simulink model "FullCarLateral"  (R2023b)
settings: Solver=FixedStepAuto  StartTime=0.0  StopTime=30  FixedStep=dt  MaxStep=0.001  RelTol=1e-3
model workspace (MAT data in the model file):
  AMU : Simulink.Signal (value not decoded)
  EPSILON : Simulink.Signal (value not decoded)
  FZO : Simulink.Signal (value not decoded)
  LCX : Simulink.Signal (value not decoded)
  LCY : Simulink.Signal (value not decoded)
  LCZ : Simulink.Signal (value not decoded)
  LEX : Simulink.Signal (value not decoded)
  LEY : Simulink.Signal (value not decoded)
  LFZO : Simulink.Signal (value not decoded)
  LHX : Simulink.Signal (value not decoded)
  LHY : Simulink.Signal (value not decoded)
  LKXKAPPA : Simulink.Signal (value not decoded)
  LKYALPHA : Simulink.Signal (value not decoded)
  LKYGAMMA : Simulink.Signal (value not decoded)
  LKZGAMMA : Simulink.Signal (value not decoded)
  LMR : Simulink.Signal (value not decoded)
  LMUV : Simulink.Signal (value not decoded)
  LMUX : Simulink.Signal (value not decoded)
  LMUXAST : Simulink.Signal (value not decoded)
  LMUXPRIME : Simulink.Signal (value not decoded)
  LMUY : Simulink.Signal (value not decoded)
  LMUYAST : Simulink.Signal (value not decoded)
  LMUYPRIME : Simulink.Signal (value not decoded)
  LMX : Simulink.Signal (value not decoded)
  LMY : Simulink.Signal (value not decoded)
  LS : Simulink.Signal (value not decoded)
  LT : Simulink.Signal (value not decoded)
  LVX : Simulink.Signal (value not decoded)
  LVY : Simulink.Signal (value not decoded)
  LVYKAPPA : Simulink.Signal (value not decoded)
  LXALPHA : Simulink.Signal (value not decoded)
  LYKAPPA : Simulink.Signal (value not decoded)
  PCX1 : Simulink.Signal (value not decoded)
  PCY1 : Simulink.Signal (value not decoded)
  PDX1 : Simulink.Signal (value not decoded)
  PDX2 : Simulink.Signal (value not decoded)
  PDX3 : Simulink.Signal (value not decoded)
  PDY1 : Simulink.Signal (value not decoded)
  PDY2 : Simulink.Signal (value not decoded)
  PDY3 : Simulink.Signal (value not decoded)
  PEX1 : Simulink.Signal (value not decoded)
  PEX2 : Simulink.Signal (value not decoded)
  PEX3 : Simulink.Signal (value not decoded)
  PEX4 : Simulink.Signal (value not decoded)
  PEY1 : Simulink.Signal (value not decoded)
  PEY2 : Simulink.Signal (value not decoded)
  PEY3 : Simulink.Signal (value not decoded)
  PEY4 : Simulink.Signal (value not decoded)
  PEY5 : Simulink.Signal (value not decoded)
  PHX1 : Simulink.Signal (value not decoded)
  PHX2 : Simulink.Signal (value not decoded)
  PHY1 : Simulink.Signal (value not decoded)
  PHY2 : Simulink.Signal (value not decoded)
  PKX1 : Simulink.Signal (value not decoded)
  PKX2 : Simulink.Signal (value not decoded)
  PKX3 : Simulink.Signal (value not decoded)
  PKY1 : Simulink.Signal (value not decoded)
  PKY2 : Simulink.Signal (value not decoded)
  PKY3 : Simulink.Signal (value not decoded)
  PKY4 : Simulink.Signal (value not decoded)
  PKY5 : Simulink.Signal (value not decoded)
  PKY6 : Simulink.Signal (value not decoded)
  PKY7 : Simulink.Signal (value not decoded)
  PVX1 : Simulink.Signal (value not decoded)
  PVX2 : Simulink.Signal (value not decoded)
  PVY1 : Simulink.Signal (value not decoded)
  PVY2 : Simulink.Signal (value not decoded)
  PVY3 : Simulink.Signal (value not decoded)
  PVY4 : Simulink.Signal (value not decoded)
  QBZ1 : Simulink.Signal (value not decoded)
  QBZ10 : Simulink.Signal (value not decoded)
  QBZ2 : Simulink.Signal (value not decoded)
  QBZ3 : Simulink.Signal (value not decoded)
  QBZ5 : Simulink.Signal (value not decoded)
  QBZ6 : Simulink.Signal (value not decoded)
  QBZ9 : Simulink.Signal (value not decoded)
  QCZ1 : Simulink.Signal (value not decoded)
  QDZ1 : Simulink.Signal (value not decoded)
  QDZ10 : Simulink.Signal (value not decoded)
  QDZ11 : Simulink.Signal (value not decoded)
  QDZ2 : Simulink.Signal (value not decoded)
  QDZ3 : Simulink.Signal (value not decoded)
  QDZ4 : Simulink.Signal (value not decoded)
  QDZ6 : Simulink.Signal (value not decoded)
  QDZ7 : Simulink.Signal (value not decoded)
  QDZ8 : Simulink.Signal (value not decoded)
  QDZ9 : Simulink.Signal (value not decoded)
  QEZ1 : Simulink.Signal (value not decoded)
  QEZ2 : Simulink.Signal (value not decoded)
  QEZ3 : Simulink.Signal (value not decoded)
  QEZ4 : Simulink.Signal (value not decoded)
  QEZ5 : Simulink.Signal (value not decoded)
  QHZ1 : Simulink.Signal (value not decoded)
  QHZ2 : Simulink.Signal (value not decoded)
  QHZ3 : Simulink.Signal (value not decoded)
  QHZ4 : Simulink.Signal (value not decoded)
  QSX1 : Simulink.Signal (value not decoded)
  QSX2 : Simulink.Signal (value not decoded)
  QSX3 : Simulink.Signal (value not decoded)
  QX1 : Simulink.Signal (value not decoded)
  QX2 : Simulink.Signal (value not decoded)
  QX3 : Simulink.Signal (value not decoded)
  QX4 : Simulink.Signal (value not decoded)
  QX5 : Simulink.Signal (value not decoded)
  QX6 : Simulink.Signal (value not decoded)
  RBX1 : Simulink.Signal (value not decoded)
  RBX2 : Simulink.Signal (value not decoded)
  RBX3 : Simulink.Signal (value not decoded)
  RBY1 : Simulink.Signal (value not decoded)
  RBY2 : Simulink.Signal (value not decoded)
  RBY3 : Simulink.Signal (value not decoded)
  RBY4 : Simulink.Signal (value not decoded)
  RCX1 : Simulink.Signal (value not decoded)
  RCY1 : Simulink.Signal (value not decoded)
  REX1 : Simulink.Signal (value not decoded)
  REX2 : Simulink.Signal (value not decoded)
  REY1 : Simulink.Signal (value not decoded)
  REY2 : Simulink.Signal (value not decoded)
  RHX1 : Simulink.Signal (value not decoded)
  RHY1 : Simulink.Signal (value not decoded)
  RHY2 : Simulink.Signal (value not decoded)
  RO : Simulink.Signal (value not decoded)
  RVY1 : Simulink.Signal (value not decoded)
  RVY2 : Simulink.Signal (value not decoded)
  RVY3 : Simulink.Signal (value not decoded)
  RVY4 : Simulink.Signal (value not decoded)
  RVY5 : Simulink.Signal (value not decoded)
  RVY6 : Simulink.Signal (value not decoded)
  SSZ1 : Simulink.Signal (value not decoded)
  SSZ2 : Simulink.Signal (value not decoded)
  SSZ3 : Simulink.Signal (value not decoded)
  SSZ4 : Simulink.Signal (value not decoded)
  VCX : Simulink.Signal (value not decoded)
  ZETA0 : Simulink.Signal (value not decoded)
  ZETA1 : Simulink.Signal (value not decoded)
  ZETA2 : Simulink.Signal (value not decoded)
  ZETA3 : Simulink.Signal (value not decoded)
  ZETA4 : Simulink.Signal (value not decoded)
  ZETA5 : Simulink.Signal (value not decoded)
  ZETA6 : Simulink.Signal (value not decoded)
  ZETA7 : Simulink.Signal (value not decoded)
  ZETA8 : Simulink.Signal (value not decoded)
values from neighbouring files (symbols this model uses):
  A = load('PSS LATERAL FORCE COEFFS.mat').A    [FullCarLateralParams.m]
  B = load('PSS ALIGNING TORQUE COEFFS.mat').B    [FullCarLateralParams.m]
  b = 0.085    [FullCarLateralParams.m]
  C = load('COMBINED OVERTURNING MOMENT COEFFS.mat').C    [FullCarLateralParams.m]
  c_roll = 0.1    [FullCarLateralParams.m]
  cD = 1.23    [FullCarLateralParams.m]
  cL = 3.71    [FullCarLateralParams.m]
  D = load('PLS LONGITUDINAL FORCE COEFFS.mat').D    [FullCarLateralParams.m]
  dt = 0.001    [FullCarLateralParams.m]
  E = load('COMBINED LONGITUDINAL FORCE COEFFS.mat').E    [FullCarLateralParams.m]
  e_FL = atan(tf/lf)    [FullCarLateralParams.m]
  e_FR = atan(lf/tf)    [FullCarLateralParams.m]
  e_RL = atan(lr/tr)    [FullCarLateralParams.m]
  e_RR = atan(tr/lr)    [FullCarLateralParams.m]
  F = load('COMBINED LATERAL FORCE COEFFS.mat').F    [FullCarLateralParams.m]
  frontalA = 1    [FullCarLateralParams.m]
  g = 9.81    [FullCarLateralParams.m]
  G = load('COMBINED ALIGNING TORQUE COEFFS.mat').G    [FullCarLateralParams.m]
  gearboxEff = 0.95    [FullCarLateralParams.m]
  GR = 11.86    [FullCarLateralParams.m]
  hCG = 0.2    [FullCarLateralParams.m]
  Ix_wheel = (0.07829 + Ix_motor*GR*GR) * Ix_wheel_factor    (= 0.1168307304)    [FullCarLateralParams.m]
  Iz_vehicle = 125    [FullCarLateralParams.m]
  lf = wb - lr    (= 0.755)    [FullCarLateralParams.m]
  lowpassT = 0.05    [FullCarLateralParams.m]
  lr = 0.78    [FullCarLateralParams.m]
  m = 250    [FullCarLateralParams.m]
  motorOmegaLimit = 2094    [FullCarLateralParams.m]
  R_FL = sqrt(tf^2 + lf^2)    [FullCarLateralParams.m]
  R_FR = R_FL    [FullCarLateralParams.m]
  R_RL = sqrt(tr^2 + lr^2)    [FullCarLateralParams.m]
  R_RR = R_RL    [FullCarLateralParams.m]
  R_wheel = 0.2    [FullCarLateralParams.m]
  rho = 1.293    [FullCarLateralParams.m]
  tireFactor_X_Accel = 0.6    [FullCarLateralParams.m]
  tireFactor_X_Brake = 0.6    [FullCarLateralParams.m]
  tireFactor_Y = 1    [FullCarLateralParams.m]
  TLLTD = 0.5    [FullCarLateralParams.m]
  tr = trackWidth / 2    (= 0.6)    [FullCarLateralParams.m]
  trackWidth = 1.2    [FullCarLateralParams.m]
  wb = 1.535    [FullCarLateralParams.m]
  wheelSideBrakeFactor = 1    [FullCarLateralParams.m]
undefined symbols (not defined in the file or in its folder): trackReference
libraries: simulink_extras x11, eeGeneralControl x3, slpidlib x2, simulink x2
(part 4 of 6)

== system FullCarLateral/Car/Wheel Dynamics/Subsystem7/Accel. or Rolling No Slip ==
  Requested Motor Torque : Inport
  FX Resistance : Inport  Port=2
  Long Corner Vel : Inport  Port=3
  Action Port : ActionPort  ActionPortLabel=if(u1 >= 0)
  Accelerating : Subsystem  TreatAsAtomicUnit=on
  If : If  IfExpression=u1 > rollingNoSlipTorqueThreshold
  Merge : Merge
  Merge1 : Merge
  Rolling No Slip : Subsystem  TreatAsAtomicUnit=on
  Wheel Omega : Outport
  Constrained Motor Torque : Outport  Port=2
  wires:
  Merge1/1 -> Constrained Motor Torque/1
  Rolling No Slip/2(Constrained Motor Torque) -> Merge1/2
  Accelerating/2(Constrained Motor Torque) -> Merge1/1
  FX Resistance/1 -> Accelerating/2(FX Resistance)
  Long Corner Vel/1 -> Rolling No Slip/1(Long Corner Vel)
  Merge/1 -> Wheel Omega/1
  Rolling No Slip/1(No Slip Wheel Omega) -> Merge/2
  Accelerating/1(Accelerating Wheel Omega) -> Merge/1
  If/2 -> Rolling No Slip/Action
  If/1 -> Accelerating/Action
  Requested Motor Torque/1 -> If/1, Rolling No Slip/2(Requested Motor Torque), Accelerating/1(Requested Motor Torque)

== system FullCarLateral/Car/Wheel Dynamics/Subsystem7/Braking ==
  Requested Motor Torque : Inport
  FX Resistance : Inport  Port=2
  Action Port : ActionPort  ActionPortLabel=else
  Constant : Constant  Value=0
  Motor Omega Calc : Subsystem
  Switch : Switch  Criteria=u2 > Threshold  SaturateOnIntegerOverflow=off  InputSameDT=off
  Wheel Omega : Outport
  Constrained Motor Torque : Outport  Port=2
  wires:
  Constant/1 -> Switch/3
  Switch/1 -> Wheel Omega/1
  Motor Omega Calc/1(Wheel Omega) -> Switch/1, Switch/2
  FX Resistance/1 -> Motor Omega Calc/2(FX Resistance)
  Requested Motor Torque/1 -> Motor Omega Calc/1(Motor Torque), Constrained Motor Torque/1

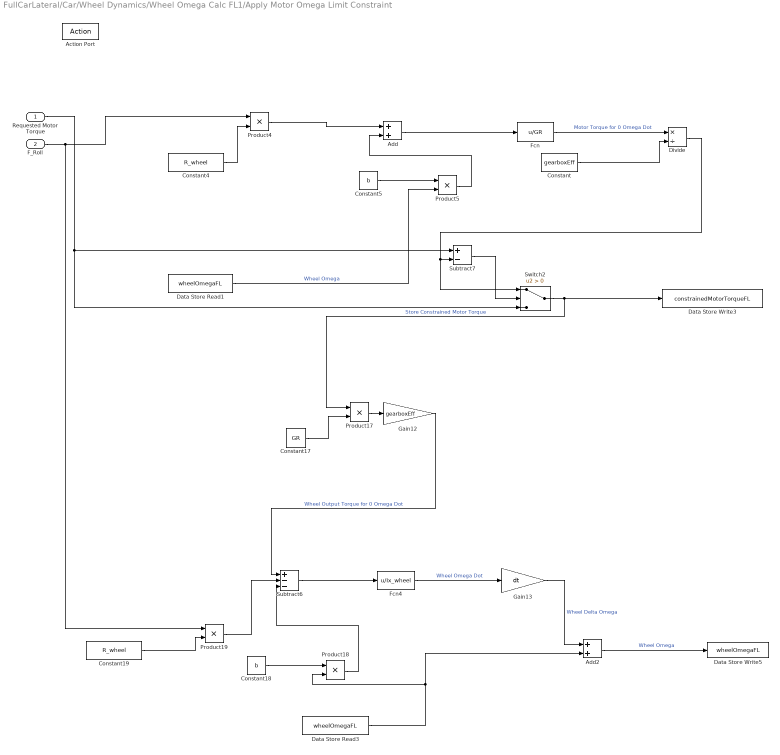
== system FullCarLateral/Car/Wheel Dynamics/Wheel Omega Calc FL1/Apply Motor Omega Limit Constraint ==
  Requested Motor Torque : Inport
  F_Roll : Inport  Port=2
  Action Port : ActionPort
  Add : Sum
  Add2 : Sum
  Constant : Constant  Value=gearboxEff
  Constant17 : Constant  Value=GR
  Constant18 : Constant  Value=b
  Constant19 : Constant  Value=R_wheel
  Constant4 : Constant  Value=R_wheel
  Constant5 : Constant  Value=b
  Data Store Read1 : DataStoreRead  DataStoreName=wheelOmegaFL  IndexOptions=Index vector (dialog)  Indices=1  OutputSizes=1
  Data Store Read3 : DataStoreRead  DataStoreName=wheelOmegaFL  IndexOptions=Index vector (dialog)  Indices=1  OutputSizes=1
  Data Store Write3 : DataStoreWrite  DataStoreName=constrainedMotorTorqueFL  IndexOptions=Index vector (dialog)  Indices=1  OutputSizes=1
  Data Store Write5 : DataStoreWrite  DataStoreName=wheelOmegaFL  IndexOptions=Index vector (dialog)  Indices=1  OutputSizes=1
  Divide : Product  Inputs=*/
  Fcn : Fcn  Expr=u/GR
  Fcn4 : Fcn  Expr=u/Ix_wheel
  Gain12 : Gain  Gain=gearboxEff
  Gain13 : Gain  Gain=dt
  Product{4..5,17..19} (5 alike) : Product
  Subtract6 : Sum  Inputs=+--
  Subtract7 : Sum  Inputs=+-
  Switch2 : Switch  Criteria=u2 > Threshold  SaturateOnIntegerOverflow=off  InputSameDT=off
  wires:
  Constant5/1 -> Product5/1
  Add/1 -> Fcn/1
  Constant4/1 -> Product4/2
  Product5/1 -> Add/2
  Product4/1 -> Add/1
  Switch2/1 -> Product17/1, Data Store Write3/1  "Store Constrained Motor Torque"
  Gain12/1 -> Subtract6/1  "Wheel Output Torque for 0 Omega Dot"
  Subtract7/1 -> Switch2/2
  Data Store Read3/1 -> Add2/2, Product18/2
  Constant18/1 -> Product18/1
  Requested Motor Torque/1 -> Subtract7/1, Switch2/3
  Product17/1 -> Gain12/1
  Fcn4/1 -> Gain13/1  "Wheel Omega Dot"
  Subtract6/1 -> Fcn4/1
  Product19/1 -> Subtract6/2
  Constant17/1 -> Product17/2
  Gain13/1 -> Add2/1  "Wheel Delta Omega"
  Product18/1 -> Subtract6/3
  Add2/1 -> Data Store Write5/1  "Wheel Omega"
  Constant19/1 -> Product19/2
  F_Roll/1 -> Product19/1, Product4/1
  Data Store Read1/1 -> Product5/2  "Wheel Omega"
  Fcn/1 -> Divide/1  "Motor Torque for 0 Omega Dot"
  Constant/1 -> Divide/2
  Divide/1 -> Switch2/1, Subtract7/2

== system FullCarLateral/Car/Wheel Dynamics/Wheel Omega Calc FL1/No Omega Limit Constraint ==
  Wheel Omega : Inport
  Unconstrained Requested Motor Torque : Inport  Port=2
  Action Port : ActionPort
  Constant1 : Constant  Value=0
  Data Store Write3 : DataStoreWrite  DataStoreName=constrainedMotorTorqueFL  IndexOptions=Index vector (dialog)  Indices=1  OutputSizes=1
  Data Store Write6 : DataStoreWrite  DataStoreName=wheelOmegaFL  IndexOptions=Index vector (dialog)  Indices=1  OutputSizes=1
  Switch : Switch  Criteria=u2 > Threshold  SaturateOnIntegerOverflow=off  InputSameDT=off
  wires:
  Unconstrained Requested Motor Torque/1 -> Data Store Write3/1
  Constant1/1 -> Switch/3
  Wheel Omega/1 -> Switch/1, Switch/2  "Wheel Omega"
  Switch/1 -> Data Store Write6/1

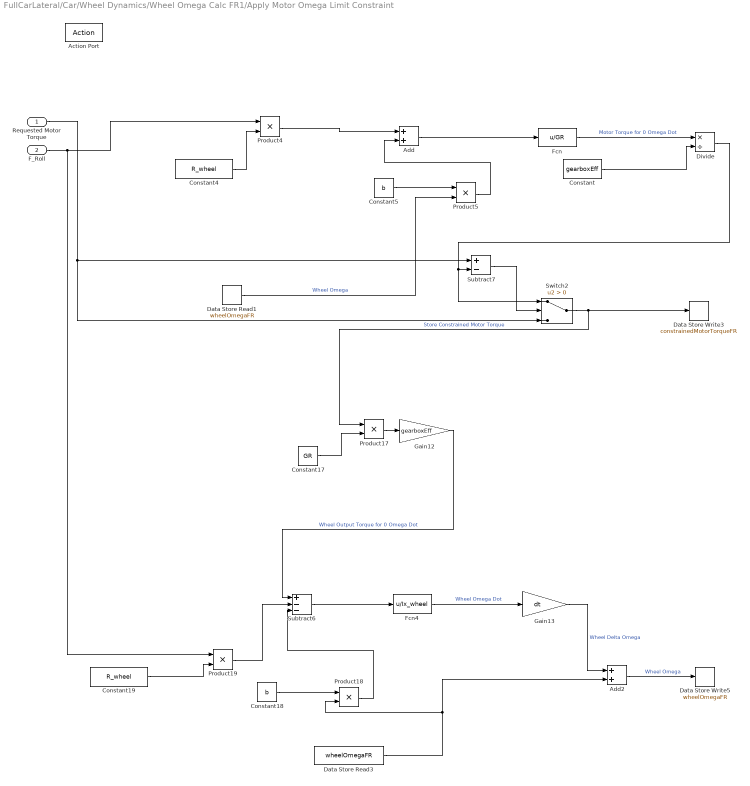
== system FullCarLateral/Car/Wheel Dynamics/Wheel Omega Calc FR1/Apply Motor Omega Limit Constraint ==
  Requested Motor Torque : Inport
  F_Roll : Inport  Port=2
  Action Port : ActionPort
  Add : Sum
  Add2 : Sum
  Constant : Constant  Value=gearboxEff
  Constant17 : Constant  Value=GR
  Constant18 : Constant  Value=b
  Constant19 : Constant  Value=R_wheel
  Constant4 : Constant  Value=R_wheel
  Constant5 : Constant  Value=b
  Data Store Read1 : DataStoreRead  DataStoreName=wheelOmegaFR  IndexOptions=Index vector (dialog)  Indices=1  OutputSizes=1
  Data Store Read3 : DataStoreRead  DataStoreName=wheelOmegaFR  IndexOptions=Index vector (dialog)  Indices=1  OutputSizes=1
  Data Store Write3 : DataStoreWrite  DataStoreName=constrainedMotorTorqueFR  IndexOptions=Index vector (dialog)  Indices=1  OutputSizes=1
  Data Store Write5 : DataStoreWrite  DataStoreName=wheelOmegaFR  IndexOptions=Index vector (dialog)  Indices=1  OutputSizes=1
  Divide : Product  Inputs=*/
  Fcn : Fcn  Expr=u/GR
  Fcn4 : Fcn  Expr=u/Ix_wheel
  Gain12 : Gain  Gain=gearboxEff
  Gain13 : Gain  Gain=dt
  Product{4..5,17..19} (5 alike) : Product
  Subtract6 : Sum  Inputs=+--
  Subtract7 : Sum  Inputs=+-
  Switch2 : Switch  Criteria=u2 > Threshold  SaturateOnIntegerOverflow=off  InputSameDT=off
  wires:
  Divide/1 -> Subtract7/2, Switch2/1
  Constant/1 -> Divide/2
  Fcn/1 -> Divide/1  "Motor Torque for 0 Omega Dot"
  Data Store Read1/1 -> Product5/2  "Wheel Omega"
  F_Roll/1 -> Product4/1, Product19/1
  Constant19/1 -> Product19/2
  Add2/1 -> Data Store Write5/1  "Wheel Omega"
  Product18/1 -> Subtract6/3
  Gain13/1 -> Add2/1  "Wheel Delta Omega"
  Constant17/1 -> Product17/2
  Product19/1 -> Subtract6/2
  Subtract6/1 -> Fcn4/1
  Fcn4/1 -> Gain13/1  "Wheel Omega Dot"
  Product17/1 -> Gain12/1
  Requested Motor Torque/1 -> Switch2/3, Subtract7/1
  Constant18/1 -> Product18/1
  Data Store Read3/1 -> Product18/2, Add2/2
  Subtract7/1 -> Switch2/2
  Gain12/1 -> Subtract6/1  "Wheel Output Torque for 0 Omega Dot"
  Switch2/1 -> Data Store Write3/1, Product17/1  "Store Constrained Motor Torque"
  Product4/1 -> Add/1
  Product5/1 -> Add/2
  Constant4/1 -> Product4/2
  Add/1 -> Fcn/1
  Constant5/1 -> Product5/1

== system FullCarLateral/Car/Wheel Dynamics/Wheel Omega Calc FR1/No Omega Limit Constraint ==
  Wheel Omega : Inport
  Unconstrained Requested Motor Torque : Inport  Port=2
  Action Port : ActionPort
  Constant1 : Constant  Value=0
  Data Store Write3 : DataStoreWrite  DataStoreName=constrainedMotorTorqueFR  IndexOptions=Index vector (dialog)  Indices=1  OutputSizes=1
  Data Store Write6 : DataStoreWrite  DataStoreName=wheelOmegaFR  IndexOptions=Index vector (dialog)  Indices=1  OutputSizes=1
  Switch : Switch  Criteria=u2 > Threshold  SaturateOnIntegerOverflow=off  InputSameDT=off
  wires:
  Unconstrained Requested Motor Torque/1 -> Data Store Write3/1
  Switch/1 -> Data Store Write6/1
  Wheel Omega/1 -> Switch/2, Switch/1  "Wheel Omega"
  Constant1/1 -> Switch/3

== system FullCarLateral/Car/Wheel Dynamics/Wheel Omega Calc RL1/Apply Motor Omega Limit Constraint ==
  Requested Motor Torque : Inport
  F_Roll : Inport  Port=2
  Action Port : ActionPort
  Add : Sum
  Add2 : Sum
  Constant : Constant  Value=gearboxEff
  Constant17 : Constant  Value=GR
  Constant18 : Constant  Value=b
  Constant19 : Constant  Value=R_wheel
  Constant4 : Constant  Value=R_wheel
  Constant5 : Constant  Value=b
  Data Store Read1 : DataStoreRead  DataStoreName=wheelOmegaRL  IndexOptions=Index vector (dialog)  Indices=1  OutputSizes=1
  Data Store Read3 : DataStoreRead  DataStoreName=wheelOmegaRL  IndexOptions=Index vector (dialog)  Indices=1  OutputSizes=1
  Data Store Write3 : DataStoreWrite  DataStoreName=constrainedMotorTorqueRL  IndexOptions=Index vector (dialog)  Indices=1  OutputSizes=1
  Data Store Write5 : DataStoreWrite  DataStoreName=wheelOmegaRL  IndexOptions=Index vector (dialog)  Indices=1  OutputSizes=1
  Divide : Product  Inputs=*/
  Fcn : Fcn  Expr=u/GR
  Fcn4 : Fcn  Expr=u/Ix_wheel
  Gain12 : Gain  Gain=gearboxEff
  Gain13 : Gain  Gain=dt
  Product{4..5,17..19} (5 alike) : Product
  Subtract6 : Sum  Inputs=+--
  Subtract7 : Sum  Inputs=+-
  Switch2 : Switch  Criteria=u2 > Threshold  SaturateOnIntegerOverflow=off  InputSameDT=off
  wires:
  Constant5/1 -> Product5/1
  Add/1 -> Fcn/1
  Constant4/1 -> Product4/2
  Product5/1 -> Add/2
  Product4/1 -> Add/1
  Switch2/1 -> Product17/1, Data Store Write3/1  "Store Constrained Motor Torque"
  Gain12/1 -> Subtract6/1  "Wheel Output Torque for 0 Omega Dot"
  Subtract7/1 -> Switch2/2
  Data Store Read3/1 -> Add2/2, Product18/2
  Constant18/1 -> Product18/1
  Requested Motor Torque/1 -> Subtract7/1, Switch2/3
  Product17/1 -> Gain12/1
  Fcn4/1 -> Gain13/1  "Wheel Omega Dot"
  Subtract6/1 -> Fcn4/1
  Product19/1 -> Subtract6/2
  Constant17/1 -> Product17/2
  Gain13/1 -> Add2/1  "Wheel Delta Omega"
  Product18/1 -> Subtract6/3
  Add2/1 -> Data Store Write5/1  "Wheel Omega"
  Constant19/1 -> Product19/2
  F_Roll/1 -> Product19/1, Product4/1
  Data Store Read1/1 -> Product5/2  "Wheel Omega"
  Fcn/1 -> Divide/1  "Motor Torque for 0 Omega Dot"
  Constant/1 -> Divide/2
  Divide/1 -> Switch2/1, Subtract7/2

== system FullCarLateral/Car/Wheel Dynamics/Wheel Omega Calc RL1/No Omega Limit Constraint ==
  Wheel Omega : Inport
  Unconstrained Requested Motor Torque : Inport  Port=2
  Action Port : ActionPort
  Constant1 : Constant  Value=0
  Data Store Write3 : DataStoreWrite  DataStoreName=constrainedMotorTorqueRL  IndexOptions=Index vector (dialog)  Indices=1  OutputSizes=1
  Data Store Write6 : DataStoreWrite  DataStoreName=wheelOmegaRL  IndexOptions=Index vector (dialog)  Indices=1  OutputSizes=1
  Switch : Switch  Criteria=u2 > Threshold  SaturateOnIntegerOverflow=off  InputSameDT=off
  wires:
  Unconstrained Requested Motor Torque/1 -> Data Store Write3/1
  Wheel Omega/1 -> Switch/1, Switch/2  "Wheel Omega"
  Constant1/1 -> Switch/3
  Switch/1 -> Data Store Write6/1

== system FullCarLateral/Car/Wheel Dynamics/Wheel Omega Calc RR1/Apply Motor Omega Limit Constraint ==
  Requested Motor Torque : Inport
  F_Roll : Inport  Port=2
  Action Port : ActionPort
  Add : Sum
  Add2 : Sum
  Constant : Constant  Value=gearboxEff
  Constant17 : Constant  Value=GR
  Constant18 : Constant  Value=b
  Constant19 : Constant  Value=R_wheel
  Constant4 : Constant  Value=R_wheel
  Constant5 : Constant  Value=b
  Data Store Read1 : DataStoreRead  DataStoreName=wheelOmegaRR  IndexOptions=Index vector (dialog)  Indices=1  OutputSizes=1
  Data Store Read3 : DataStoreRead  DataStoreName=wheelOmegaRR  IndexOptions=Index vector (dialog)  Indices=1  OutputSizes=1
  Data Store Write3 : DataStoreWrite  DataStoreName=constrainedMotorTorqueRR  IndexOptions=Index vector (dialog)  Indices=1  OutputSizes=1
  Data Store Write5 : DataStoreWrite  DataStoreName=wheelOmegaRR  IndexOptions=Index vector (dialog)  Indices=1  OutputSizes=1
  Divide : Product  Inputs=*/
  Fcn : Fcn  Expr=u/GR
  Fcn4 : Fcn  Expr=u/Ix_wheel
  Gain12 : Gain  Gain=gearboxEff
  Gain13 : Gain  Gain=dt
  Product{4..5,17..19} (5 alike) : Product
  Subtract6 : Sum  Inputs=+--
  Subtract7 : Sum  Inputs=+-
  Switch2 : Switch  Criteria=u2 > Threshold  SaturateOnIntegerOverflow=off  InputSameDT=off
  wires:
  Divide/1 -> Subtract7/2, Switch2/1
  Constant/1 -> Divide/2
  Fcn/1 -> Divide/1  "Motor Torque for 0 Omega Dot"
  Data Store Read1/1 -> Product5/2  "Wheel Omega"
  F_Roll/1 -> Product4/1, Product19/1
  Constant19/1 -> Product19/2
  Add2/1 -> Data Store Write5/1  "Wheel Omega"
  Product18/1 -> Subtract6/3
  Gain13/1 -> Add2/1  "Wheel Delta Omega"
  Constant17/1 -> Product17/2
  Product19/1 -> Subtract6/2
  Subtract6/1 -> Fcn4/1
  Fcn4/1 -> Gain13/1  "Wheel Omega Dot"
  Product17/1 -> Gain12/1
  Requested Motor Torque/1 -> Switch2/3, Subtract7/1
  Constant18/1 -> Product18/1
  Data Store Read3/1 -> Product18/2, Add2/2
  Subtract7/1 -> Switch2/2
  Gain12/1 -> Subtract6/1  "Wheel Output Torque for 0 Omega Dot"
  Switch2/1 -> Data Store Write3/1, Product17/1  "Store Constrained Motor Torque"
  Product4/1 -> Add/1
  Product5/1 -> Add/2
  Constant4/1 -> Product4/2
  Add/1 -> Fcn/1
  Constant5/1 -> Product5/1

== system FullCarLateral/Car/Wheel Dynamics/Wheel Omega Calc RR1/No Omega Limit Constraint ==
  Wheel Omega : Inport
  Unconstrained Requested Motor Torque : Inport  Port=2
  Action Port : ActionPort
  Constant1 : Constant  Value=0
  Data Store Write3 : DataStoreWrite  DataStoreName=constrainedMotorTorqueRR  IndexOptions=Index vector (dialog)  Indices=1  OutputSizes=1
  Data Store Write6 : DataStoreWrite  DataStoreName=wheelOmegaRR  IndexOptions=Index vector (dialog)  Indices=1  OutputSizes=1
  Switch : Switch  Criteria=u2 > Threshold  SaturateOnIntegerOverflow=off  InputSameDT=off
  wires:
  Unconstrained Requested Motor Torque/1 -> Data Store Write3/1
  Constant1/1 -> Switch/3
  Wheel Omega/1 -> Switch/1, Switch/2
  Switch/1 -> Data Store Write6/1

== system FullCarLateral/Car/Wheel Dynamics/Subsystem4/Accel. or Rolling No Slip/Accelerating ==
  Requested Motor Torque : Inport
  FX Resistance : Inport  Port=2
  Action Port : ActionPort  ActionPortLabel=if(u1 > rollingNoSlipTorqueThreshold)
  Constrain Torque and Recalculate Omega : Subsystem  TreatAsAtomicUnit=on
  Gain : Gain  Gain=GR
  If : If  IfExpression=u1 > motorOmegaLimit
  If Action Subsystem1 : Subsystem  TreatAsAtomicUnit=on
  Merge : Merge
  Merge1 : Merge
  Motor Omega Calc : Subsystem
  Accelerating Wheel Omega : Outport
  Constrained Motor Torque : Outport  Port=2
  wires:
  If/1 -> Constrain Torque and Recalculate Omega/Action
  Requested Motor Torque/1 -> If Action Subsystem1/2(Requested Motor Torque), Motor Omega Calc/1(Motor Torque)
  FX Resistance/1 -> Constrain Torque and Recalculate Omega/2(FX Resistance), Motor Omega Calc/2(FX Resistance)
  Motor Omega Calc/1(Wheel Omega) -> Constrain Torque and Recalculate Omega/1(Wheel Omega), If Action Subsystem1/1(Unconstrained Wheel Omega), Gain/1
  Gain/1 -> If/1  "Motor Omega"
  If/2 -> If Action Subsystem1/Action
  Constrain Torque and Recalculate Omega/1(Constrained Wheel Omega) -> Merge/1
  If Action Subsystem1/1(Constrained Wheel Omega) -> Merge/2
  Merge/1 -> Motor Omega Calc/3(Prev. Wheel Omega), Accelerating Wheel Omega/1
  Constrain Torque and Recalculate Omega/2(Constrained Motor Torque) -> Merge1/1
  If Action Subsystem1/2(Constrained Motor Torque) -> Merge1/2
  Merge1/1 -> Constrained Motor Torque/1

== system FullCarLateral/Car/Wheel Dynamics/Subsystem4/Accel. or Rolling No Slip/Rolling No Slip ==
  Long Corner Vel : Inport
  Requested Motor Torque : Inport  Port=2
  Action Port : ActionPort  ActionPortLabel=else
  Abs : Abs  SaturateOnIntegerOverflow=off
  Constant : Constant  Value=R_wheel
  Divide : Product  Inputs=*/
  No Slip Wheel Omega : Outport
  Constrained Motor Torque : Outport  Port=2
  wires:
  Long Corner Vel/1 -> Abs/1
  Constant/1 -> Divide/2
  Divide/1 -> No Slip Wheel Omega/1
  Requested Motor Torque/1 -> Constrained Motor Torque/1
  Abs/1 -> Divide/1

== system FullCarLateral/Car/Wheel Dynamics/Subsystem4/Braking/Motor Omega Calc ==
  Motor Torque : Inport
  FX Resistance : Inport  Port=2
  Add2 : Sum  Inputs=+--
  Add3 : Sum
  Constant4 : Constant  Value=Ix_wheel
  Constant5 : Constant  Value=dt
  Constant6 : Constant  Value=GR
  Constant7 : Constant  Value=R_wheel
  Divide1 : Product  Inputs=*/
  Gain3 : Gain  Gain=gearboxEff
  Gain5 : Gain  Gain=b
  Memory1 : Memory
  Product3 : Product
  Product4 : Product
  Product5 : Product
  Wheel Omega : Outport
  wires:
  Constant7/1 -> Product4/2
  Add3/1 -> Memory1/1
  Product4/1 -> Add2/2  "Resistive Torque From FX Resistance"
  Divide1/1 -> Product5/1  "dWheel Omega dt"
  Gain5/1 -> Add2/3
  Memory1/1 -> Wheel Omega/1, Add3/2, Gain5/1  "Wheel Omega"
  Gain3/1 -> Add2/1  "Requested Wheel Side Torque"
  Product3/1 -> Gain3/1
  Product5/1 -> Add3/1  "dWheel Omega"
  Constant5/1 -> Product5/2
  Add2/1 -> Divide1/1
  Constant4/1 -> Divide1/2
  Constant6/1 -> Product3/2
  FX Resistance/1 -> Product4/1
  Motor Torque/1 -> Product3/1

== system FullCarLateral/Car/Wheel Dynamics/Subsystem5/Accel. or Rolling No Slip/Accelerating ==
  Requested Motor Torque : Inport
  FX Resistance : Inport  Port=2
  Action Port : ActionPort  ActionPortLabel=if(u1 > rollingNoSlipTorqueThreshold)
  Constrain Torque and Recalculate Omega : Subsystem  TreatAsAtomicUnit=on
  Gain : Gain  Gain=GR
  If : If  IfExpression=u1 > motorOmegaLimit
  If Action Subsystem1 : Subsystem  TreatAsAtomicUnit=on
  Merge : Merge
  Merge1 : Merge
  Motor Omega Calc : Subsystem
  Accelerating Wheel Omega : Outport
  Constrained Motor Torque : Outport  Port=2
  wires:
  Merge1/1 -> Constrained Motor Torque/1
  If Action Subsystem1/2(Constrained Motor Torque) -> Merge1/2
  Constrain Torque and Recalculate Omega/2(Constrained Motor Torque) -> Merge1/1
  Merge/1 -> Accelerating Wheel Omega/1, Motor Omega Calc/3(Prev. Wheel Omega)
  If Action Subsystem1/1(Constrained Wheel Omega) -> Merge/2
  Constrain Torque and Recalculate Omega/1(Constrained Wheel Omega) -> Merge/1
  If/2 -> If Action Subsystem1/Action
  Gain/1 -> If/1  "Motor Omega"
  Motor Omega Calc/1(Wheel Omega) -> Gain/1, If Action Subsystem1/1(Unconstrained Wheel Omega), Constrain Torque and Recalculate Omega/1(Wheel Omega)
  FX Resistance/1 -> Motor Omega Calc/2(FX Resistance), Constrain Torque and Recalculate Omega/2(FX Resistance)
  Requested Motor Torque/1 -> Motor Omega Calc/1(Motor Torque), If Action Subsystem1/2(Requested Motor Torque)
  If/1 -> Constrain Torque and Recalculate Omega/Action

== system FullCarLateral/Car/Wheel Dynamics/Subsystem5/Accel. or Rolling No Slip/Rolling No Slip ==
  Long Corner Vel : Inport
  Requested Motor Torque : Inport  Port=2
  Action Port : ActionPort  ActionPortLabel=else
  Abs : Abs  SaturateOnIntegerOverflow=off
  Constant : Constant  Value=R_wheel
  Divide : Product  Inputs=*/
  No Slip Wheel Omega : Outport
  Constrained Motor Torque : Outport  Port=2
  wires:
  Long Corner Vel/1 -> Abs/1
  Constant/1 -> Divide/2
  Divide/1 -> No Slip Wheel Omega/1
  Requested Motor Torque/1 -> Constrained Motor Torque/1
  Abs/1 -> Divide/1

== system FullCarLateral/Car/Wheel Dynamics/Subsystem5/Braking/Motor Omega Calc ==
  Motor Torque : Inport
  FX Resistance : Inport  Port=2
  Add2 : Sum  Inputs=+--
  Add3 : Sum
  Constant4 : Constant  Value=Ix_wheel
  Constant5 : Constant  Value=dt
  Constant6 : Constant  Value=GR
  Constant7 : Constant  Value=R_wheel
  Divide1 : Product  Inputs=*/
  Gain3 : Gain  Gain=gearboxEff
  Gain5 : Gain  Gain=b
  Memory1 : Memory
  Product3 : Product
  Product4 : Product
  Product5 : Product
  Wheel Omega : Outport
  wires:
  Motor Torque/1 -> Product3/1
  FX Resistance/1 -> Product4/1
  Constant6/1 -> Product3/2
  Constant4/1 -> Divide1/2
  Add2/1 -> Divide1/1
  Constant5/1 -> Product5/2
  Product5/1 -> Add3/1  "dWheel Omega"
  Product3/1 -> Gain3/1
  Gain3/1 -> Add2/1  "Requested Wheel Side Torque"
  Memory1/1 -> Gain5/1, Add3/2, Wheel Omega/1  "Wheel Omega"
  Gain5/1 -> Add2/3
  Divide1/1 -> Product5/1  "dWheel Omega dt"
  Product4/1 -> Add2/2  "Resistive Torque From FX Resistance"
  Add3/1 -> Memory1/1
  Constant7/1 -> Product4/2

== system FullCarLateral/Car/Wheel Dynamics/Subsystem6/Accel. or Rolling No Slip/Accelerating ==
  Requested Motor Torque : Inport
  FX Resistance : Inport  Port=2
  Action Port : ActionPort  ActionPortLabel=if(u1 > rollingNoSlipTorqueThreshold)
  Constrain Torque and Recalculate Omega : Subsystem  TreatAsAtomicUnit=on
  Gain : Gain  Gain=GR
  If : If  IfExpression=u1 > motorOmegaLimit
  If Action Subsystem1 : Subsystem  TreatAsAtomicUnit=on
  Merge : Merge
  Merge1 : Merge
  Motor Omega Calc : Subsystem
  Accelerating Wheel Omega : Outport
  Constrained Motor Torque : Outport  Port=2
  wires:
  If/1 -> Constrain Torque and Recalculate Omega/Action
  Requested Motor Torque/1 -> If Action Subsystem1/2(Requested Motor Torque), Motor Omega Calc/1(Motor Torque)
  FX Resistance/1 -> Constrain Torque and Recalculate Omega/2(FX Resistance), Motor Omega Calc/2(FX Resistance)
  Motor Omega Calc/1(Wheel Omega) -> Constrain Torque and Recalculate Omega/1(Wheel Omega), If Action Subsystem1/1(Unconstrained Wheel Omega), Gain/1
  Gain/1 -> If/1  "Motor Omega"
  If/2 -> If Action Subsystem1/Action
  Constrain Torque and Recalculate Omega/1(Constrained Wheel Omega) -> Merge/1
  If Action Subsystem1/1(Constrained Wheel Omega) -> Merge/2
  Merge/1 -> Motor Omega Calc/3(Prev. Wheel Omega), Accelerating Wheel Omega/1
  Constrain Torque and Recalculate Omega/2(Constrained Motor Torque) -> Merge1/1
  If Action Subsystem1/2(Constrained Motor Torque) -> Merge1/2
  Merge1/1 -> Constrained Motor Torque/1

== system FullCarLateral/Car/Wheel Dynamics/Subsystem6/Accel. or Rolling No Slip/Rolling No Slip ==
  Long Corner Vel : Inport
  Requested Motor Torque : Inport  Port=2
  Action Port : ActionPort  ActionPortLabel=else
  Abs : Abs  SaturateOnIntegerOverflow=off
  Constant : Constant  Value=R_wheel
  Divide : Product  Inputs=*/
  No Slip Wheel Omega : Outport
  Constrained Motor Torque : Outport  Port=2
  wires:
  Long Corner Vel/1 -> Abs/1
  Constant/1 -> Divide/2
  Divide/1 -> No Slip Wheel Omega/1
  Requested Motor Torque/1 -> Constrained Motor Torque/1
  Abs/1 -> Divide/1

== system FullCarLateral/Car/Wheel Dynamics/Subsystem6/Braking/Motor Omega Calc ==
  Motor Torque : Inport
  FX Resistance : Inport  Port=2
  Add2 : Sum  Inputs=+--
  Add3 : Sum
  Constant4 : Constant  Value=Ix_wheel
  Constant5 : Constant  Value=dt
  Constant6 : Constant  Value=GR
  Constant7 : Constant  Value=R_wheel
  Divide1 : Product  Inputs=*/
  Gain3 : Gain  Gain=gearboxEff
  Gain5 : Gain  Gain=b
  Memory1 : Memory
  Product3 : Product
  Product4 : Product
  Product5 : Product
  Wheel Omega : Outport
  wires:
  Constant7/1 -> Product4/2
  Add3/1 -> Memory1/1
  Product4/1 -> Add2/2  "Resistive Torque From FX Resistance"
  Divide1/1 -> Product5/1  "dWheel Omega dt"
  Gain5/1 -> Add2/3
  Memory1/1 -> Wheel Omega/1, Add3/2, Gain5/1  "Wheel Omega"
  Gain3/1 -> Add2/1  "Requested Wheel Side Torque"
  Product3/1 -> Gain3/1
  Product5/1 -> Add3/1  "dWheel Omega"
  Constant5/1 -> Product5/2
  Add2/1 -> Divide1/1
  Constant4/1 -> Divide1/2
  Constant6/1 -> Product3/2
  FX Resistance/1 -> Product4/1
  Motor Torque/1 -> Product3/1

== system FullCarLateral/Car/Wheel Dynamics/Subsystem7/Accel. or Rolling No Slip/Accelerating ==
  Requested Motor Torque : Inport
  FX Resistance : Inport  Port=2
  Action Port : ActionPort  ActionPortLabel=if(u1 > rollingNoSlipTorqueThreshold)
  Constrain Torque and Recalculate Omega : Subsystem  TreatAsAtomicUnit=on
  Gain : Gain  Gain=GR
  If : If  IfExpression=u1 > motorOmegaLimit
  If Action Subsystem1 : Subsystem  TreatAsAtomicUnit=on
  Merge : Merge
  Merge1 : Merge
  Motor Omega Calc : Subsystem
  Accelerating Wheel Omega : Outport
  Constrained Motor Torque : Outport  Port=2
  wires:
  Merge1/1 -> Constrained Motor Torque/1
  If Action Subsystem1/2(Constrained Motor Torque) -> Merge1/2
  Constrain Torque and Recalculate Omega/2(Constrained Motor Torque) -> Merge1/1
  Merge/1 -> Accelerating Wheel Omega/1, Motor Omega Calc/3(Prev. Wheel Omega)
  If Action Subsystem1/1(Constrained Wheel Omega) -> Merge/2
  Constrain Torque and Recalculate Omega/1(Constrained Wheel Omega) -> Merge/1
  If/2 -> If Action Subsystem1/Action
  Gain/1 -> If/1  "Motor Omega"
  Motor Omega Calc/1(Wheel Omega) -> Gain/1, If Action Subsystem1/1(Unconstrained Wheel Omega), Constrain Torque and Recalculate Omega/1(Wheel Omega)
  FX Resistance/1 -> Motor Omega Calc/2(FX Resistance), Constrain Torque and Recalculate Omega/2(FX Resistance)
  Requested Motor Torque/1 -> Motor Omega Calc/1(Motor Torque), If Action Subsystem1/2(Requested Motor Torque)
  If/1 -> Constrain Torque and Recalculate Omega/Action

== system FullCarLateral/Car/Wheel Dynamics/Subsystem7/Accel. or Rolling No Slip/Rolling No Slip ==
  Long Corner Vel : Inport
  Requested Motor Torque : Inport  Port=2
  Action Port : ActionPort  ActionPortLabel=else
  Abs : Abs  SaturateOnIntegerOverflow=off
  Constant : Constant  Value=R_wheel
  Divide : Product  Inputs=*/
  No Slip Wheel Omega : Outport
  Constrained Motor Torque : Outport  Port=2
  wires:
  Long Corner Vel/1 -> Abs/1
  Constant/1 -> Divide/2
  Divide/1 -> No Slip Wheel Omega/1
  Requested Motor Torque/1 -> Constrained Motor Torque/1
  Abs/1 -> Divide/1

== system FullCarLateral/Car/Wheel Dynamics/Subsystem7/Braking/Motor Omega Calc ==
  Motor Torque : Inport
  FX Resistance : Inport  Port=2
  Add2 : Sum  Inputs=+--
  Add3 : Sum
  Constant4 : Constant  Value=Ix_wheel
  Constant5 : Constant  Value=dt
  Constant6 : Constant  Value=GR
  Constant7 : Constant  Value=R_wheel
  Divide1 : Product  Inputs=*/
  Gain3 : Gain  Gain=gearboxEff
  Gain5 : Gain  Gain=b
  Memory1 : Memory
  Product3 : Product
  Product4 : Product
  Product5 : Product
  Wheel Omega : Outport
  wires:
  Motor Torque/1 -> Product3/1
  FX Resistance/1 -> Product4/1
  Constant6/1 -> Product3/2
  Constant4/1 -> Divide1/2
  Add2/1 -> Divide1/1
  Constant5/1 -> Product5/2
  Product5/1 -> Add3/1  "dWheel Omega"
  Product3/1 -> Gain3/1
  Gain3/1 -> Add2/1  "Requested Wheel Side Torque"
  Memory1/1 -> Gain5/1, Add3/2, Wheel Omega/1  "Wheel Omega"
  Gain5/1 -> Add2/3
  Divide1/1 -> Product5/1  "dWheel Omega dt"
  Product4/1 -> Add2/2  "Resistive Torque From FX Resistance"
  Add3/1 -> Memory1/1
  Constant7/1 -> Product4/2

== system FullCarLateral/Car/Wheel Dynamics/Subsystem4/Accel. or Rolling No Slip/Accelerating/Constrain Torque and Recalculate Omega ==
  Wheel Omega : Inport
  FX Resistance : Inport  Port=2
  Action Port : ActionPort  ActionPortLabel=if(u1 > motorOmegaLimit)
  Add : Sum
  Constant : Constant  Value=GR
  Constant1 : Constant  Value=motorOmegaLimit
  Constant2 : Constant  Value=GR
  Divide : Product  Inputs=*/
  Divide1 : Product  Inputs=*/
  Gain : Gain  Gain=b
  Gain1 : Gain  Gain=R_wheel
  Constrained Wheel Omega : Outport
  Constrained Motor Torque : Outport  Port=2
  wires:
  Wheel Omega/1 -> Gain/1
  Gain/1 -> Add/1
  FX Resistance/1 -> Gain1/1
  Add/1 -> Divide/1
  Constant/1 -> Divide/2
  Divide/1 -> Constrained Motor Torque/1  "Motor Torque for 0 Omega Dot"
  Gain1/1 -> Add/2
  Constant1/1 -> Divide1/1
  Constant2/1 -> Divide1/2
  Divide1/1 -> Constrained Wheel Omega/1

== system FullCarLateral/Car/Wheel Dynamics/Subsystem4/Accel. or Rolling No Slip/Accelerating/If Action Subsystem1 ==
  Unconstrained Wheel Omega : Inport
  Requested Motor Torque : Inport  Port=2
  Action Port : ActionPort  ActionPortLabel=else
  Constrained Wheel Omega : Outport
  Constrained Motor Torque : Outport  Port=2
  wires:
  Unconstrained Wheel Omega/1 -> Constrained Wheel Omega/1
  Requested Motor Torque/1 -> Constrained Motor Torque/1

== system FullCarLateral/Car/Wheel Dynamics/Subsystem4/Accel. or Rolling No Slip/Accelerating/Motor Omega Calc ==
  Motor Torque : Inport
  FX Resistance : Inport  Port=2
  Prev. Wheel Omega : Inport  Port=3
  Add2 : Sum  Inputs=+--
  Add3 : Sum
  Constant4 : Constant  Value=Ix_wheel
  Constant5 : Constant  Value=dt
  Constant6 : Constant  Value=GR
  Constant7 : Constant  Value=R_wheel
  Divide1 : Product  Inputs=*/
  Gain3 : Gain  Gain=gearboxEff
  Gain5 : Gain  Gain=b
  Memory : Memory
  Product3 : Product
  Product4 : Product
  Product5 : Product
  Wheel Omega : Outport
  wires:
  Constant7/1 -> Product4/2
  Product4/1 -> Add2/2  "Resistive Torque From FX Resistance"
  Divide1/1 -> Product5/1  "dWheel Omega dt"
  Gain5/1 -> Add2/3
  Add3/1 -> Memory/1  "Wheel Omega"
  Gain3/1 -> Add2/1  "Requested Wheel Side Torque"
  Product3/1 -> Gain3/1
  Product5/1 -> Add3/1  "dWheel Omega"
  Constant5/1 -> Product5/2
  Add2/1 -> Divide1/1
  Constant4/1 -> Divide1/2
  Constant6/1 -> Product3/2
  FX Resistance/1 -> Product4/1
  Motor Torque/1 -> Product3/1
  Prev. Wheel Omega/1 -> Add3/2, Gain5/1
  Memory/1 -> Wheel Omega/1

== system FullCarLateral/Car/Wheel Dynamics/Subsystem5/Accel. or Rolling No Slip/Accelerating/Constrain Torque and Recalculate Omega ==
  Wheel Omega : Inport
  FX Resistance : Inport  Port=2
  Action Port : ActionPort  ActionPortLabel=if(u1 > motorOmegaLimit)
  Add : Sum
  Constant : Constant  Value=GR
  Constant1 : Constant  Value=motorOmegaLimit
  Constant2 : Constant  Value=GR
  Divide : Product  Inputs=*/
  Divide1 : Product  Inputs=*/
  Gain : Gain  Gain=b
  Gain1 : Gain  Gain=R_wheel
  Constrained Wheel Omega : Outport
  Constrained Motor Torque : Outport  Port=2
  wires:
  Divide1/1 -> Constrained Wheel Omega/1
  Constant2/1 -> Divide1/2
  Constant1/1 -> Divide1/1
  Gain1/1 -> Add/2
  Divide/1 -> Constrained Motor Torque/1  "Motor Torque for 0 Omega Dot"
  Constant/1 -> Divide/2
  Add/1 -> Divide/1
  FX Resistance/1 -> Gain1/1
  Gain/1 -> Add/1
  Wheel Omega/1 -> Gain/1

== system FullCarLateral/Car/Wheel Dynamics/Subsystem5/Accel. or Rolling No Slip/Accelerating/If Action Subsystem1 ==
  Unconstrained Wheel Omega : Inport
  Requested Motor Torque : Inport  Port=2
  Action Port : ActionPort  ActionPortLabel=else
  Constrained Wheel Omega : Outport
  Constrained Motor Torque : Outport  Port=2
  wires:
  Requested Motor Torque/1 -> Constrained Motor Torque/1
  Unconstrained Wheel Omega/1 -> Constrained Wheel Omega/1

== system FullCarLateral/Car/Wheel Dynamics/Subsystem5/Accel. or Rolling No Slip/Accelerating/Motor Omega Calc ==
  Motor Torque : Inport
  FX Resistance : Inport  Port=2
  Prev. Wheel Omega : Inport  Port=3
  Add2 : Sum  Inputs=+--
  Add3 : Sum
  Constant4 : Constant  Value=Ix_wheel
  Constant5 : Constant  Value=dt
  Constant6 : Constant  Value=GR
  Constant7 : Constant  Value=R_wheel
  Divide1 : Product  Inputs=*/
  Gain3 : Gain  Gain=gearboxEff
  Gain5 : Gain  Gain=b
  Memory : Memory
  Product3 : Product
  Product4 : Product
  Product5 : Product
  Wheel Omega : Outport
  wires:
  Memory/1 -> Wheel Omega/1
  Prev. Wheel Omega/1 -> Gain5/1, Add3/2
  Motor Torque/1 -> Product3/1
  FX Resistance/1 -> Product4/1
  Constant6/1 -> Product3/2
  Constant4/1 -> Divide1/2
  Add2/1 -> Divide1/1
  Constant5/1 -> Product5/2
  Product5/1 -> Add3/1  "dWheel Omega"
  Product3/1 -> Gain3/1
  Gain3/1 -> Add2/1  "Requested Wheel Side Torque"
  Add3/1 -> Memory/1  "Wheel Omega"
  Gain5/1 -> Add2/3
  Divide1/1 -> Product5/1  "dWheel Omega dt"
  Product4/1 -> Add2/2  "Resistive Torque From FX Resistance"
  Constant7/1 -> Product4/2

== system FullCarLateral/Car/Wheel Dynamics/Subsystem6/Accel. or Rolling No Slip/Accelerating/Constrain Torque and Recalculate Omega ==
  Wheel Omega : Inport
  FX Resistance : Inport  Port=2
  Action Port : ActionPort  ActionPortLabel=if(u1 > motorOmegaLimit)
  Add : Sum
  Constant : Constant  Value=GR
  Constant1 : Constant  Value=motorOmegaLimit
  Constant2 : Constant  Value=GR
  Divide : Product  Inputs=*/
  Divide1 : Product  Inputs=*/
  Gain : Gain  Gain=b
  Gain1 : Gain  Gain=R_wheel
  Constrained Wheel Omega : Outport
  Constrained Motor Torque : Outport  Port=2
  wires:
  Wheel Omega/1 -> Gain/1
  Gain/1 -> Add/1
  FX Resistance/1 -> Gain1/1
  Add/1 -> Divide/1
  Constant/1 -> Divide/2
  Divide/1 -> Constrained Motor Torque/1  "Motor Torque for 0 Omega Dot"
  Gain1/1 -> Add/2
  Constant1/1 -> Divide1/1
  Constant2/1 -> Divide1/2
  Divide1/1 -> Constrained Wheel Omega/1

== system FullCarLateral/Car/Wheel Dynamics/Subsystem6/Accel. or Rolling No Slip/Accelerating/If Action Subsystem1 ==
  Unconstrained Wheel Omega : Inport
  Requested Motor Torque : Inport  Port=2
  Action Port : ActionPort  ActionPortLabel=else
  Constrained Wheel Omega : Outport
  Constrained Motor Torque : Outport  Port=2
  wires:
  Unconstrained Wheel Omega/1 -> Constrained Wheel Omega/1
  Requested Motor Torque/1 -> Constrained Motor Torque/1

== system FullCarLateral/Car/Wheel Dynamics/Subsystem6/Accel. or Rolling No Slip/Accelerating/Motor Omega Calc ==
  Motor Torque : Inport
  FX Resistance : Inport  Port=2
  Prev. Wheel Omega : Inport  Port=3
  Add2 : Sum  Inputs=+--
  Add3 : Sum
  Constant4 : Constant  Value=Ix_wheel
  Constant5 : Constant  Value=dt
  Constant6 : Constant  Value=GR
  Constant7 : Constant  Value=R_wheel
  Divide1 : Product  Inputs=*/
  Gain3 : Gain  Gain=gearboxEff
  Gain5 : Gain  Gain=b
  Memory : Memory
  Product3 : Product
  Product4 : Product
  Product5 : Product
  Wheel Omega : Outport
  wires:
  Constant7/1 -> Product4/2
  Product4/1 -> Add2/2  "Resistive Torque From FX Resistance"
  Divide1/1 -> Product5/1  "dWheel Omega dt"
  Gain5/1 -> Add2/3
  Add3/1 -> Memory/1  "Wheel Omega"
  Gain3/1 -> Add2/1  "Requested Wheel Side Torque"
  Product3/1 -> Gain3/1
  Product5/1 -> Add3/1  "dWheel Omega"
  Constant5/1 -> Product5/2
  Add2/1 -> Divide1/1
  Constant4/1 -> Divide1/2
  Constant6/1 -> Product3/2
  FX Resistance/1 -> Product4/1
  Motor Torque/1 -> Product3/1
  Prev. Wheel Omega/1 -> Add3/2, Gain5/1
  Memory/1 -> Wheel Omega/1

== system FullCarLateral/Car/Wheel Dynamics/Subsystem7/Accel. or Rolling No Slip/Accelerating/Constrain Torque and Recalculate Omega ==
  Wheel Omega : Inport
  FX Resistance : Inport  Port=2
  Action Port : ActionPort  ActionPortLabel=if(u1 > motorOmegaLimit)
  Add : Sum
  Constant : Constant  Value=GR
  Constant1 : Constant  Value=motorOmegaLimit
  Constant2 : Constant  Value=GR
  Divide : Product  Inputs=*/
  Divide1 : Product  Inputs=*/
  Gain : Gain  Gain=b
  Gain1 : Gain  Gain=R_wheel
  Constrained Wheel Omega : Outport
  Constrained Motor Torque : Outport  Port=2
  wires:
  Divide1/1 -> Constrained Wheel Omega/1
  Constant2/1 -> Divide1/2
  Constant1/1 -> Divide1/1
  Gain1/1 -> Add/2
  Divide/1 -> Constrained Motor Torque/1  "Motor Torque for 0 Omega Dot"
  Constant/1 -> Divide/2
  Add/1 -> Divide/1
  FX Resistance/1 -> Gain1/1
  Gain/1 -> Add/1
  Wheel Omega/1 -> Gain/1

== system FullCarLateral/Car/Wheel Dynamics/Subsystem7/Accel. or Rolling No Slip/Accelerating/If Action Subsystem1 ==
  Unconstrained Wheel Omega : Inport
  Requested Motor Torque : Inport  Port=2
  Action Port : ActionPort  ActionPortLabel=else
  Constrained Wheel Omega : Outport
  Constrained Motor Torque : Outport  Port=2
  wires:
  Requested Motor Torque/1 -> Constrained Motor Torque/1
  Unconstrained Wheel Omega/1 -> Constrained Wheel Omega/1

== system FullCarLateral/Car/Wheel Dynamics/Subsystem7/Accel. or Rolling No Slip/Accelerating/Motor Omega Calc ==
  Motor Torque : Inport
  FX Resistance : Inport  Port=2
  Prev. Wheel Omega : Inport  Port=3
  Add2 : Sum  Inputs=+--
  Add3 : Sum
  Constant4 : Constant  Value=Ix_wheel
  Constant5 : Constant  Value=dt
  Constant6 : Constant  Value=GR
  Constant7 : Constant  Value=R_wheel
  Divide1 : Product  Inputs=*/
  Gain3 : Gain  Gain=gearboxEff
  Gain5 : Gain  Gain=b
  Memory : Memory
  Product3 : Product
  Product4 : Product
  Product5 : Product
  Wheel Omega : Outport
  wires:
  Memory/1 -> Wheel Omega/1
  Prev. Wheel Omega/1 -> Gain5/1, Add3/2
  Motor Torque/1 -> Product3/1
  FX Resistance/1 -> Product4/1
  Constant6/1 -> Product3/2
  Constant4/1 -> Divide1/2
  Add2/1 -> Divide1/1
  Constant5/1 -> Product5/2
  Product5/1 -> Add3/1  "dWheel Omega"
  Product3/1 -> Gain3/1
  Gain3/1 -> Add2/1  "Requested Wheel Side Torque"
  Add3/1 -> Memory/1  "Wheel Omega"
  Gain5/1 -> Add2/3
  Divide1/1 -> Product5/1  "dWheel Omega dt"
  Product4/1 -> Add2/2  "Resistive Torque From FX Resistance"
  Constant7/1 -> Product4/2
